simulink model "Problem2"  (R2023b)
settings: Solver=VariableStepAuto  StartTime=0.0  StopTime=t  RelTol=1e-3
values from neighbouring files (symbols this model uses):
  a = 1    [Problem2_script.m]
  am = 2    [Problem2_script.m]
  b = 5    [Problem2_script.m]
  bm = 2    [Problem2_script.m]
  gamma1 = 10    [Problem2_script.m]
  gamma2 = 10    [Problem2_script.m]
  ref = 1    [Problem2_script.m]
  Ts = 5    [Problem2_script.m]
settings Model: Creator=eliasoa  LastModifiedBy=Elias

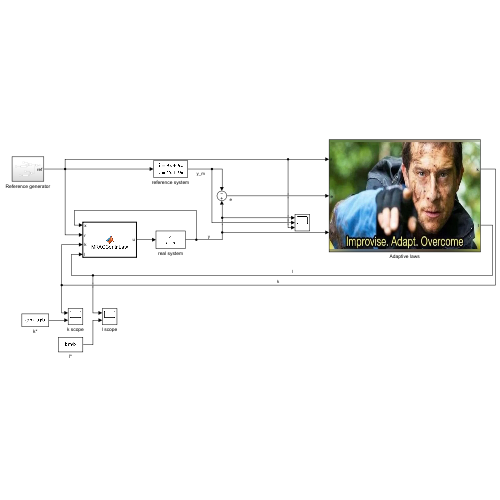
[thumbnail: Simulink's stored preview of the top-level diagram]
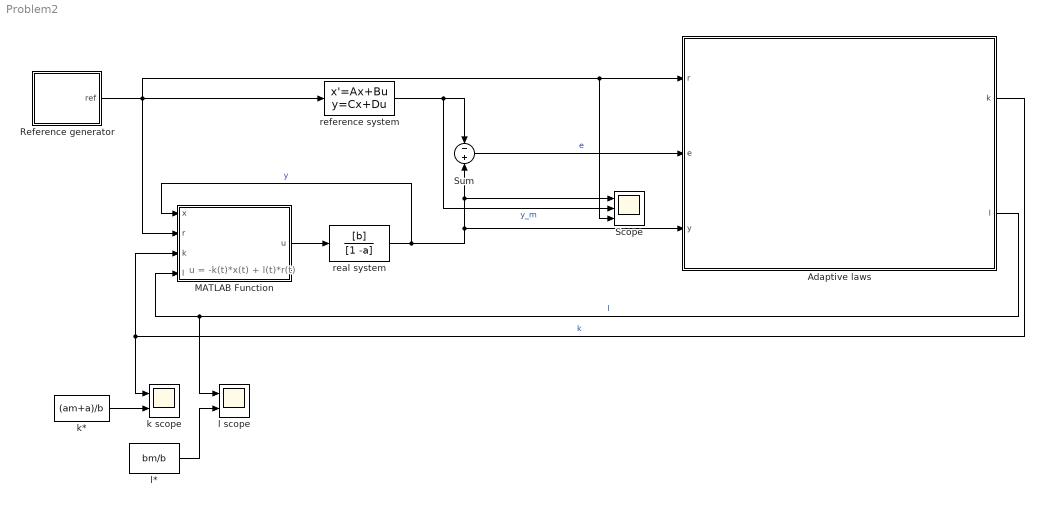
== system Problem2 ==
  note: u = -k(t)*x(t) + l(t)*r(t)
  Adaptive laws : Subsystem
      mask Display: image('improvise.png');
  MATLAB Function : MATLAB Function  TreatAsAtomicUnit=on
  Reference generator : Subsystem
  Scope : Scope  NumInputPorts=3
  Sum : Sum  Inputs=-+
  k scope : Scope  NumInputPorts=2
  k* : Constant  Value=(am+a)/b
  l scope : Scope  NumInputPorts=2
  l* : Constant  Value=bm/b
  real system : TransferFcn  Numerator=[b]  Denominator=[1 -a]
  reference system : StateSpace  A=-am  B=bm  D=0  InitialCondition=0
  wires:
  reference system/1 -> Sum/1, Scope/2  "y_m"
  MATLAB Function/1(u) -> real system/1
  real system/1 -> Adaptive laws/3(y), Scope/1, Sum/2, MATLAB Function/1(x)  "y"
  Sum/1 -> Adaptive laws/2(e)  "e"
  Adaptive laws/1(k) -> k scope/1, MATLAB Function/3(k)  "k"
  Adaptive laws/2(l) -> MATLAB Function/4(l), l scope/1  "l"
  Reference generator/1(ref) -> Scope/3, Adaptive laws/1(r), MATLAB Function/2(r), reference system/1
  k*/1 -> k scope/2
  l*/1 -> l scope/2

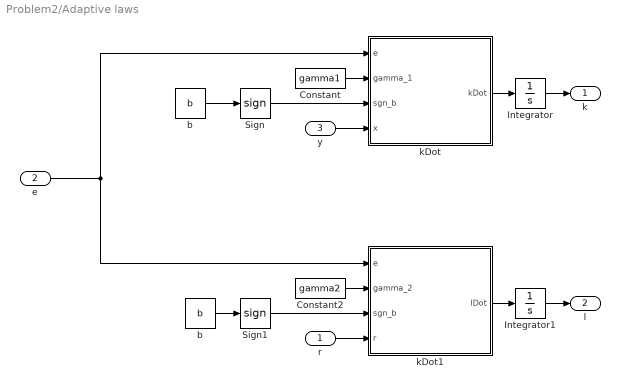
== system Problem2/Adaptive laws ==
  r : Inport
  e : Inport  Port=2
  y : Inport  Port=3
  Constant : Constant  Value=gamma1
  Constant2 : Constant  Value=gamma2
  Integrator : Integrator
  Integrator1 : Integrator
  Sign : Signum
  Sign1 : Signum
  b : Constant  Value=b
  "b " : Constant  Value=b
  kDot : MATLAB Function  TreatAsAtomicUnit=on
  kDot1 : MATLAB Function  TreatAsAtomicUnit=on
  k : Outport
  l : Outport  Port=2
  wires:
  Constant2/1 -> kDot1/2(gamma_2)
  kDot/1(kDot) -> Integrator/1
  y/1 -> kDot/4(x)
  e/1 -> kDot/1(e), kDot1/1(e)
  b/1 -> Sign/1
  Integrator1/1 -> l/1
  Constant/1 -> kDot/2(gamma_1)
  kDot1/1(lDot) -> Integrator1/1
  Sign1/1 -> kDot1/3(sgn_b)
  Sign/1 -> kDot/3(sgn_b)
  "b "/1 -> Sign1/1
  Integrator/1 -> k/1
  r/1 -> kDot1/4(r)

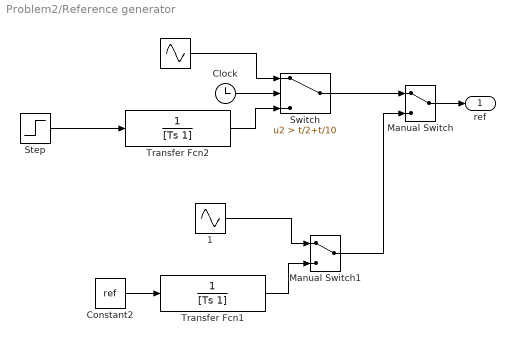
== system Problem2/Reference generator ==
  " " : Sin  SampleTime=0
  " 1" : Sin  SampleTime=0
  Clock : Clock
  Constant2 : Constant  Value=ref
  Manual Switch : ManualSwitch
  Manual Switch1 : ManualSwitch
  Step : Step  Time=t-10  After=ref  SampleTime=0
  Switch : Switch  Criteria=u2 > Threshold  Threshold=t/2+t/10  SaturateOnIntegerOverflow=off  InputSameDT=off
  Transfer Fcn1 : TransferFcn  Denominator=[Ts 1]
  Transfer Fcn2 : TransferFcn  Denominator=[Ts 1]
  ref : Outport
  wires:
  " "/1 -> Switch/1
  Step/1 -> Transfer Fcn2/1
  Clock/1 -> Switch/2
  Transfer Fcn2/1 -> Switch/3
  Manual Switch/1 -> ref/1
  Switch/1 -> Manual Switch/1
  Manual Switch1/1 -> Manual Switch/2
  " 1"/1 -> Manual Switch1/1
  Constant2/1 -> Transfer Fcn1/1
  Transfer Fcn1/1 -> Manual Switch1/2

== matlab function Problem2/Adaptive laws/kDot ==
  data: e input; gamma_1 input; sgn_b input; x input; kDot output
function kDot = kDot(e,gamma_1,sgn_b,x)

kDot = gamma_1*e*sgn_b*x;

== matlab function Problem2/MATLAB Function ==
  data: x input; u output; r input; k input; l input
function u = MRACContrlLaw(x,r,k,l)

u = -k*x + l*r;

== matlab function Problem2/Adaptive laws/kDot1 ==
  data: e input; gamma_2 input; sgn_b input; r input; lDot output
function lDot = lDot(e,gamma_2,sgn_b,r)

lDot = -gamma_2*e*sgn_b*r;
